simulink model "FrictionIdentificationImproved"  (R2013a)
settings: Solver=FixedStepDiscrete  StartTime=0.0  StopTime=60  FixedStep=0.01  RelTol=1e-3
values from neighbouring files (symbols this model uses):
  joint = CoupledJoints('experiments', 'iCubGenova03', 'torso')    [CoupledExper-IDLE.m]    (also in CoupledExper.m = joint.loadRefFile('ref'); CoupledJoints.m = [joint Motor(date,robotName, part, type,'yaw')]; JointStructure.m = struct; ReferenceLoad.m = joint.loadReference('ref'))
libraries: WBCLibrary x21, dspmtrx3 x2
settings Model: Creator=Raffaello  LastModifiedBy=Raffaello
settings DataIOCC: LimitDataPoints=off  OutputSaveName=out
settings DebuggingCC: InheritedTsInSrcMsg=none

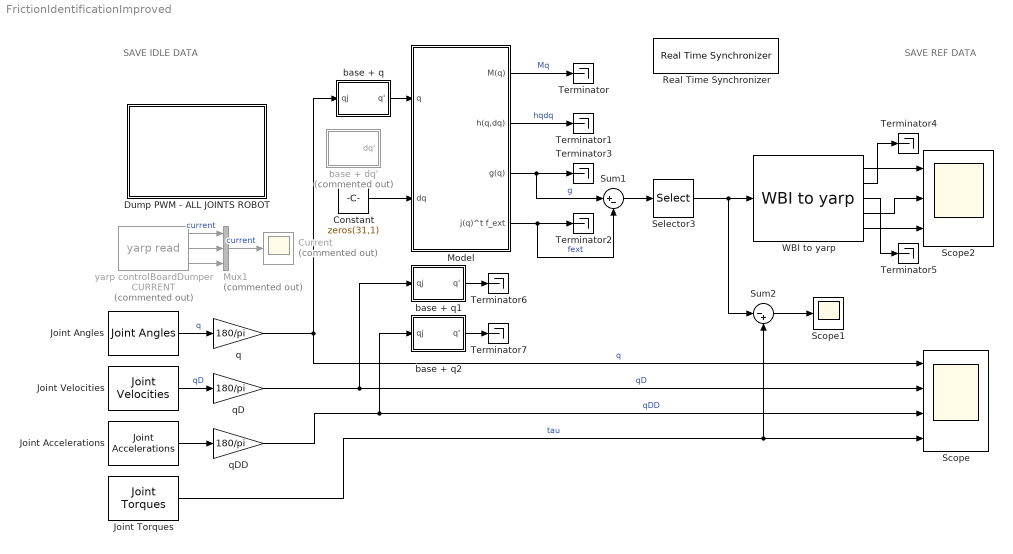
== system FrictionIdentificationImproved ==
  note: SAVE IDLE DATA
  note: SAVE REF DATA
  Constant : Constant  Value=zeros(31,1)
  Current : Scope  Commented=on
      settings: YMin=-3750  YMax=1750  SaveName=ScopeData3
  Dump PWM - ALL JOINTS ROBOT : Subsystem
  Joint Accelerations : WBCLibrary/wholeBodyStates/Joint Accelerations  robotName=robot.robotName  localName=robot.localName
  Joint Angles : WBCLibrary/wholeBodyStates/Joint Angles  robotName=robot.robotName  localName=robot.localName
  Joint Torques : WBCLibrary/wholeBodyStates/Joint Torques  robotName=robot.robotName  localName=robot.localName
  Joint Velocities : WBCLibrary/wholeBodyStates/Joint Velocities  robotName=robot.robotName  localName=robot.localName
  Model : Subsystem
  Mux1 : Mux  Commented=on  Inputs=3
  Real Time Synchronizer : WBCLibrary/Utilities/Real Time Synchronizer  Priority=-10  threadPeriod=robot.Ts
  Scope : Scope  NumInputPorts=4
      settings: ShowLegends=on  TimeRange=60  YMin=-15~-5~-20~-7  YMax=15~5~25~6  SaveName=ScopeData2
  Scope1 : Scope
      settings: YMin=-13  YMax=2  SaveName=ScopeData4
  Scope2 : Scope  NumInputPorts=3
      settings: ShowLegends=on  YMin=-5~-25~-25  YMax=1.5~2.5~2.5  SaveName=ScopeData6
  Selector3 : Selector  InputPortWidth=31  IndexOptions=Index vector (dialog)  Indices=[7:31]  OutputSizes=1
  Sum1 : Sum  Inputs=|+-
  Sum2 : Sum  Inputs=|-+
  Terminator{,1..7} (8 alike) : Terminator
  WBI to yarp : WBCLibrary/Utilities/WBI to yarp
  base + dq' : Subsystem  Commented=on
  base + q : Subsystem
  base + q1 : Subsystem
  base + q2 : Subsystem
  q : Gain  Gain=180/pi
  qD : Gain  Gain=180/pi
  qDD : Gain  Gain=180/pi
  yarp controlBoardDumper CURRENT : WBCLibrary/Utilities/yarp read  Commented=on  from=['/controlBoardDumper/' joint.group_select '/getCurrents']  to='...'  num=3  blocking=off  timestamp=off
  wires:
  Joint Angles/1 -> q/1  "q"
  Joint Velocities/1 -> qD/1  "qD"
  Joint Torques/1 -> Sum2/2, Scope/4  "tau"
  Mux1/1 -> Current/1  "current"
  Joint Accelerations/1 -> qDD/1
  qDD/1 -> base + q2/1(qj), Scope/3  "qDD"
  yarp controlBoardDumper CURRENT/1 -> Mux1/1  "current"
  yarp controlBoardDumper CURRENT/2 -> Mux1/2
  yarp controlBoardDumper CURRENT/3 -> Mux1/3
  q/1 -> Scope/1, base + q/1(qj)  "q"
  qD/1 -> base + q1/1(qj), Scope/2  "qD"
  Model/3(g(q)) -> Terminator3/1, Sum1/1  "g"
  base + q/1(q') -> Model/1(q)
  Model/1(M(q)) -> Terminator/1  "Mq"
  Model/2(h(q,dq)) -> Terminator1/1  "hqdq"
  Model/4(j(q)^t f_ext) -> Sum1/2, Terminator2/1  "fext"
  Sum1/1 -> Selector3/1
  WBI to yarp/5 -> Scope2/3
  Selector3/1 -> Sum2/1, WBI to yarp/1
  WBI to yarp/4 -> Scope2/2
  WBI to yarp/1 -> Scope2/1
  Constant/1 -> Model/2(dq)
  WBI to yarp/2 -> Terminator4/1
  WBI to yarp/3 -> Terminator5/1
  base + q2/1(q') -> Terminator7/1
  base + q1/1(q') -> Terminator6/1
  Sum2/1 -> Scope1/1

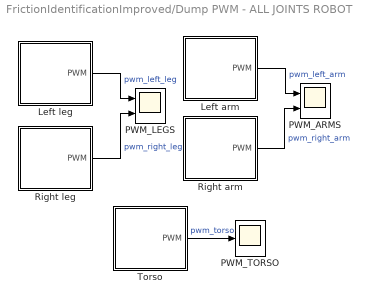
== system FrictionIdentificationImproved/Dump PWM - ALL JOINTS ROBOT ==
  Left arm : Subsystem  mask{type_arm='left_arm'}
      mask prompts: type_arm "Type leg"
  Left leg : Subsystem  mask{type_arm='left_leg'}
      mask prompts: type_arm "Type leg"
  PWM_ARMS : Scope  NumInputPorts=2
      settings: TimeRange=60  YMin=-10~-10  YMax=12.5~15
  PWM_LEGS : Scope  NumInputPorts=2
      settings: TimeRange=60  YMin=-10~-10  YMax=12.5~15
  PWM_TORSO : Scope
      settings: TimeRange=60  YMin=-10  YMax=12.5  SaveName=ScopeData5
  Right arm : Subsystem  mask{type_arm='right_arm'}
      mask prompts: type_arm "Type leg"
  Right leg : Subsystem  mask{type_arm='right_leg'}
      mask prompts: type_arm "Type leg"
  Torso : Subsystem  mask{type_arm='left_arm'}
      mask prompts: type_arm "Type leg"
  wires:
  Left arm/1(PWM) -> PWM_ARMS/1  "pwm_left_arm"
  Right arm/1(PWM) -> PWM_ARMS/2  "pwm_right_arm"
  Torso/1(PWM) -> PWM_TORSO/1  "pwm_torso"
  Right leg/1(PWM) -> PWM_LEGS/2  "pwm_right_leg"
  Left leg/1(PWM) -> PWM_LEGS/1  "pwm_left_leg"

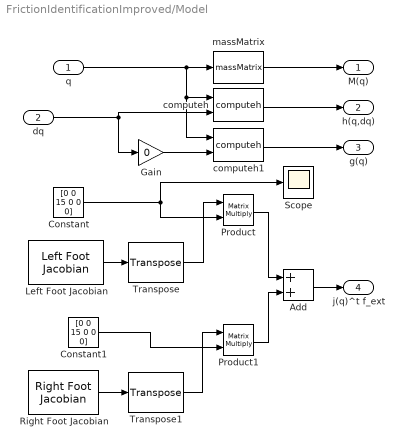
== system FrictionIdentificationImproved/Model ==
  q : Inport
  dq : Inport  Port=2
  Add : Sum
  Constant : Constant  Value=[0 0 15 0 0 0]
  Constant1 : Constant  Value=[0 0 15 0 0 0]
  Gain : Gain  Gain=0
  Left Foot Jacobian : WBCLibrary/wholeBodyModel/Jacobians/Left Foot Jacobian  robotName=robot.robotName  localName=robot.localName
  Product : Product  Multiplication=Matrix(*)
  Product1 : Product  Multiplication=Matrix(*)
  Right Foot Jacobian : WBCLibrary/wholeBodyModel/Jacobians/Right Foot Jacobian  robotName=robot.robotName  localName=robot.localName
  Scope : Scope
  Transpose : dspmtrx3/Transpose  Hermitian=off  overflowFlag=off
  Transpose1 : dspmtrx3/Transpose  Hermitian=off  overflowFlag=off
  computeh : WBCLibrary/wholeBodyModel/Dynamics/computeh  val=7  robotname=robot.robotName  localname=robot.localName
  computeh1 : WBCLibrary/wholeBodyModel/Dynamics/computeh  val=7  robotname=robot.robotName  localname=robot.localName
  massMatrix : WBCLibrary/wholeBodyModel/Dynamics/massMatrix  val=8  robotname=robot.robotName  localname=robot.localName
  M(q) : Outport
  h(q,dq) : Outport  Port=2
  g(q) : Outport  Port=3
  j(q)^t f_ext : Outport  Port=4
  wires:
  Gain/1 -> computeh1/2
  computeh1/1 -> g(q)/1
  computeh/1 -> h(q,dq)/1
  massMatrix/1 -> M(q)/1
  q/1 -> computeh1/1, computeh/1, massMatrix/1
  dq/1 -> computeh/2, Gain/1
  Left Foot Jacobian/1 -> Transpose/1
  Right Foot Jacobian/1 -> Transpose1/1
  Constant/1 -> Product/2, Scope/1
  Transpose/1 -> Product/1
  Constant1/1 -> Product1/2
  Transpose1/1 -> Product1/1
  Product/1 -> Add/1
  Product1/1 -> Add/2
  Add/1 -> j(q)^t f_ext/1

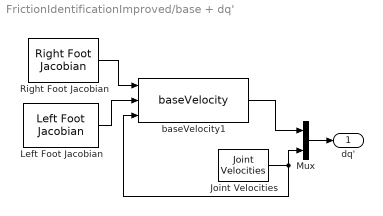
== system FrictionIdentificationImproved/base + dq' ==
  Joint Velocities : WBCLibrary/wholeBodyStates/Joint Velocities  robotName=robot.robotName  localName=robot.localName
  Left Foot Jacobian : WBCLibrary/wholeBodyModel/Jacobians/Left Foot Jacobian  robotName=robot.robotName  localName=robot.localName
  Mux : Mux  Inputs=2
  Right Foot Jacobian : WBCLibrary/wholeBodyModel/Jacobians/Right Foot Jacobian  robotName=robot.robotName  localName=robot.localName
  baseVelocity1 : WBCLibrary/Utilities/baseVelocity
  dq' : Outport
  wires:
  Left Foot Jacobian/1 -> baseVelocity1/2
  Right Foot Jacobian/1 -> baseVelocity1/1
  baseVelocity1/1 -> Mux/1
  Joint Velocities/1 -> baseVelocity1/3, Mux/2
  Mux/1 -> dq'/1

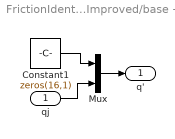
== system FrictionIdentificationImproved/base + q ==
  qj : Inport
  Constant1 : Constant  Value=zeros(16,1)
  Mux : Mux  Inputs=2
  q' : Outport
  wires:
  Mux/1 -> q'/1
  qj/1 -> Mux/2
  Constant1/1 -> Mux/1

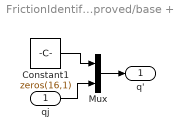
== system FrictionIdentificationImproved/base + q1 ==
  qj : Inport
  Constant1 : Constant  Value=zeros(16,1)
  Mux : Mux  Inputs=2
  q' : Outport
  wires:
  Mux/1 -> q'/1
  qj/1 -> Mux/2
  Constant1/1 -> Mux/1

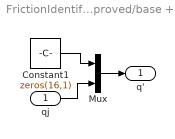
== system FrictionIdentificationImproved/base + q2 ==
  qj : Inport
  Constant1 : Constant  Value=zeros(16,1)
  Mux : Mux  Inputs=2
  q' : Outport
  wires:
  Constant1/1 -> Mux/1
  qj/1 -> Mux/2
  Mux/1 -> q'/1

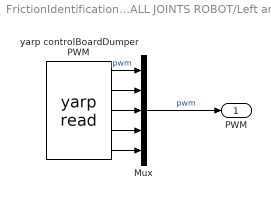
== system FrictionIdentificationImproved/Dump PWM - ALL JOINTS ROBOT/Left arm ==
  Mux : Mux  Inputs=5
  yarp controlBoardDumper PWM : WBCLibrary/Utilities/yarp read  from=['/controlBoardDumper/' type_arm '/getOutputs']  to='...'  num=5  blocking=off  timestamp=off
  PWM : Outport
  wires:
  Mux/1 -> PWM/1  "pwm"
  yarp controlBoardDumper PWM/1 -> Mux/1  "pwm"
  yarp controlBoardDumper PWM/3 -> Mux/3
  yarp controlBoardDumper PWM/2 -> Mux/2
  yarp controlBoardDumper PWM/5 -> Mux/5
  yarp controlBoardDumper PWM/4 -> Mux/4

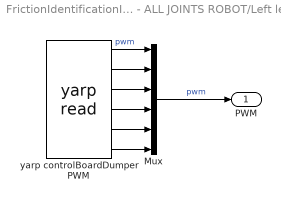
== system FrictionIdentificationImproved/Dump PWM - ALL JOINTS ROBOT/Left leg ==
  Mux : Mux  Inputs=6
  yarp controlBoardDumper PWM : WBCLibrary/Utilities/yarp read  from=['/controlBoardDumper/' type_arm '/getOutputs']  to='...'  num=6  blocking=off  timestamp=off
  PWM : Outport
  wires:
  Mux/1 -> PWM/1  "pwm"
  yarp controlBoardDumper PWM/1 -> Mux/1  "pwm"
  yarp controlBoardDumper PWM/3 -> Mux/3
  yarp controlBoardDumper PWM/2 -> Mux/2
  yarp controlBoardDumper PWM/5 -> Mux/5
  yarp controlBoardDumper PWM/6 -> Mux/6
  yarp controlBoardDumper PWM/4 -> Mux/4

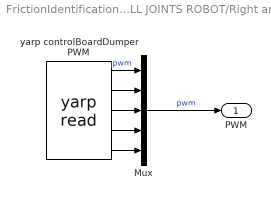
== system FrictionIdentificationImproved/Dump PWM - ALL JOINTS ROBOT/Right arm ==
  Mux : Mux  Inputs=5
  yarp controlBoardDumper PWM : WBCLibrary/Utilities/yarp read  from=['/controlBoardDumper/' type_arm '/getOutputs']  to='...'  num=5  blocking=off  timestamp=off
  PWM : Outport
  wires:
  Mux/1 -> PWM/1  "pwm"
  yarp controlBoardDumper PWM/1 -> Mux/1  "pwm"
  yarp controlBoardDumper PWM/3 -> Mux/3
  yarp controlBoardDumper PWM/2 -> Mux/2
  yarp controlBoardDumper PWM/5 -> Mux/5
  yarp controlBoardDumper PWM/4 -> Mux/4

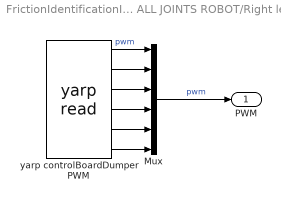
== system FrictionIdentificationImproved/Dump PWM - ALL JOINTS ROBOT/Right leg ==
  Mux : Mux  Inputs=6
  yarp controlBoardDumper PWM : WBCLibrary/Utilities/yarp read  from=['/controlBoardDumper/' type_arm '/getOutputs']  to='...'  num=6  blocking=off  timestamp=off
  PWM : Outport
  wires:
  Mux/1 -> PWM/1  "pwm"
  yarp controlBoardDumper PWM/1 -> Mux/1  "pwm"
  yarp controlBoardDumper PWM/3 -> Mux/3
  yarp controlBoardDumper PWM/2 -> Mux/2
  yarp controlBoardDumper PWM/5 -> Mux/5
  yarp controlBoardDumper PWM/6 -> Mux/6
  yarp controlBoardDumper PWM/4 -> Mux/4

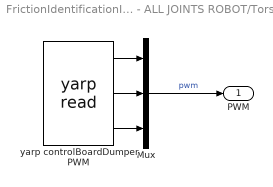
== system FrictionIdentificationImproved/Dump PWM - ALL JOINTS ROBOT/Torso ==
  Mux : Mux  Inputs=3
  yarp controlBoardDumper PWM : WBCLibrary/Utilities/yarp read  from=['/controlBoardDumper/' type_arm '/getOutputs']  to='...'  num=3  blocking=off  timestamp=off
  PWM : Outport
  wires:
  Mux/1 -> PWM/1  "pwm"
  yarp controlBoardDumper PWM/1 -> Mux/1
  yarp controlBoardDumper PWM/3 -> Mux/3
  yarp controlBoardDumper PWM/2 -> Mux/2
